simulink model "simulink_Pcontroller"  (R2016a)
settings: Solver=ode1  StartTime=0.0  StopTime=inf  FixedStep=0.1  RelTol=1e-3
undefined symbols (not defined in the file): serial
libraries: instrumentlib x4, simulink x2, dspswit3 x1
settings Model: Creator=Andrei  LastModifiedBy=Andrei

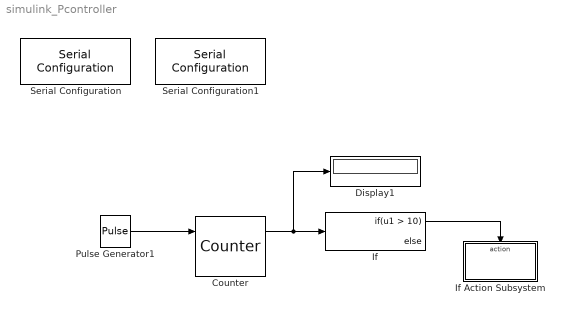
== system simulink_Pcontroller ==
  Counter : dspswit3/Counter  Direction=Up  CountEvent=Falling edge  CounterSize=8 bits  MaxCount=255  InitialCount=0  Output=Count and Hit  HitValue=32  ResetInput=on  SamplesPerFrame=1  Ts=1  CntDtype=uint8  HitDtype=Logical
  Display1 : Display
  If : If  IfExpression=u1 > 10
  If Action Subsystem : Subsystem  TreatAsAtomicUnit=on
  Pulse Generator1 : DiscretePulseGenerator  PulseType=Time based  Period=500  PulseWidth=50
  Serial Configuration : instrumentlib/Serial Configuration  Priority=-200000  ComPortMenu=COM5  ComPort=COM5  ObjConstructor=serial('COM5');  BaudRate=9600  DataBits=8  Parity=none  StopBits=1  FlowControl=none  Timeout=10  ByteOrder=LittleEndian
  Serial Configuration1 : instrumentlib/Serial Configuration  Priority=-200000  ComPortMenu=COM3  ComPort=COM3  ObjConstructor=serial('COM3');  BaudRate=38400  DataBits=8  Parity=none  StopBits=1  FlowControl=none  Timeout=10  ByteOrder=LittleEndian
  wires:
  Counter/1 -> Display1/1, If/1
  Pulse Generator1/1 -> Counter/1
  If/1 -> If Action Subsystem/Action

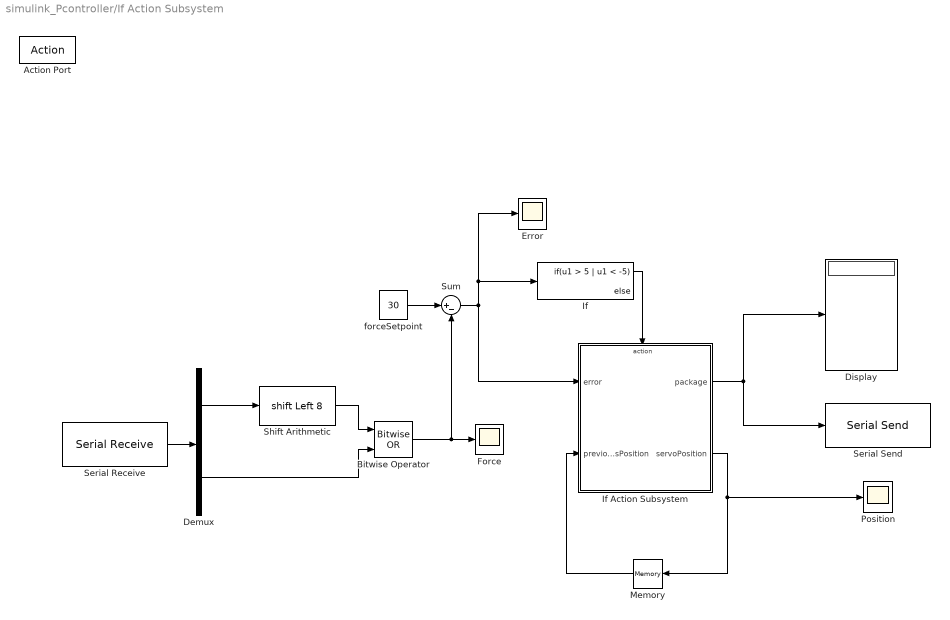
== system simulink_Pcontroller/If Action Subsystem ==
  Action Port : ActionPort  ActionType=then
  Bitwise Operator : simulink/Logic and Bit Operations/Bitwise Operator  logicop=OR  UseBitMask=off  NumInputPorts=2  BitMask=bin2dec('11011001')  BitMaskRealWorld=Stored Integer
  Demux : Demux  Outputs=2
  Display : Display
  "Error " : Scope
  Force : Scope
  If : If  IfExpression=u1 > 5 | u1 < -5
  If Action Subsystem : Subsystem  TreatAsAtomicUnit=on
  Memory : Memory  X0=512  InheritSampleTime=on
  "Position " : Scope
  Serial Receive : instrumentlib/Serial Receive  ComPortMenu=COM5  ComPort=COM5  ObjConstructor=serial('COM5');  Header=$  Terminator=!  DataSize="[1  2]"  DataType=uint8  EnableBlockingMode=on  ActionDataUnavailable=Output last received value  CustomValue=0  SampleTime=0.1
  Serial Send : instrumentlib/Serial Send  ComPortMenu=COM3  ComPort=COM3  ObjConstructor=serial('COM3');  Terminator=<none>  EnableBlockingMode=on
  Shift Arithmetic : ArithShift  BitShiftNumber=8  BitShiftDirection=Left
  Sum : Sum  Inputs=|+-
  forceSetpoint : Constant  Value=30
  wires:
  Serial Receive/1 -> Demux/1
  Demux/1 -> Shift Arithmetic/1
  Shift Arithmetic/1 -> Bitwise Operator/1
  Demux/2 -> Bitwise Operator/2
  Bitwise Operator/1 -> Force/1, Sum/2
  forceSetpoint/1 -> Sum/1
  Sum/1 -> "Error "/1, If/1, If Action Subsystem/1(error)
  If/1 -> If Action Subsystem/Action
  If Action Subsystem/1(package) -> Display/1, Serial Send/1
  If Action Subsystem/2(servoPosition) -> "Position "/1, Memory/1
  Memory/1 -> If Action Subsystem/2(previousPosition)

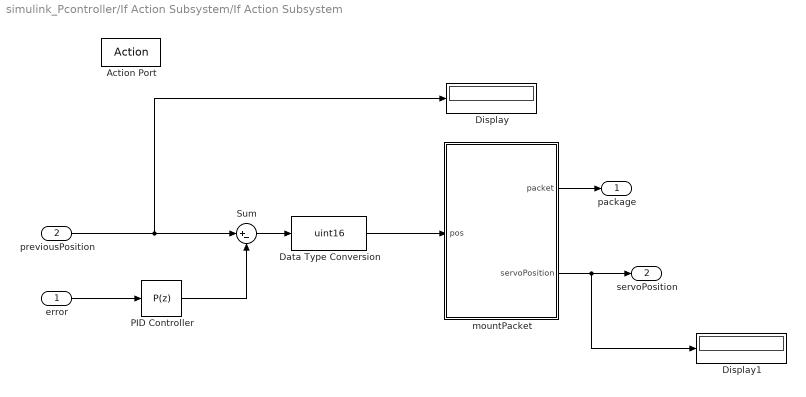
== system simulink_Pcontroller/If Action Subsystem/If Action Subsystem ==
  error : Inport
  previousPosition : Inport  Port=2
  Action Port : ActionPort  ActionType=then
  Data Type Conversion : DataTypeConversion  OutDataTypeStr=uint16
  Display : Display
  Display1 : Display
  PID Controller : simulink/Continuous/PID Controller  Controller=P  TimeDomain=Discrete-time  SampleTime=-1  IntegratorMethod=Forward Euler  FilterMethod=Forward Euler  Form=Parallel  UseFilter=on  ControllerParametersSource=internal  P=0.3  I=1  D=0  N=100  InitialConditionSource=internal  InitialConditionForIntegrator=0  InitialConditionForFilter=0  ExternalReset=none  LimitOutput=on  UpperSaturationLimit=512  LowerSaturationLimit=0  LinearizeAsGain=on  AntiWindupMode=none  Kb=1  TrackingMode=off  Kt=1  PParamMin=[]  PParamMax=[]  PParamDataTypeStr=double  IParamMin=[]  IParamMax=[]  DParamMin=[]  DParamMax=[]  NParamMin=[]  NParamMax=[]  KbParamMin=[]  KbParamMax=[]  KtParamMin=[]  KtParamMax=[]  POutMin=[]  POutMax=[]  POutDataTypeStr=double  PGainOutDataTypeStr=double  PProdOutDataTypeStr=double  IOutMin=[]  IOutMax=[]  DOutMin=[]  DOutMax=[]  NOutMin=[]  NOutMax=[]  KbOutMin=[]  KbOutMax=[]  KtOutMin=[]  KtOutMax=[]  IntegratorOutMin=[]  IntegratorOutMax=[]  FilterOutMin=[]  FilterOutMax=[]  SumOutMin=[]  SumOutMax=[]  SumI1OutMin=[]  SumI1OutMax=[]  SumI2OutMin=[]  SumI2OutMax=[]  SumI3OutMin=[]  SumI3OutMax=[]  SumDOutMin=[]  SumDOutMax=[]  SaturationOutMin=[]  SaturationOutMax=[]  SaturationOutDataTypeStr=uint16  IntegratorContinuousStateAttributes=''  IntegratorStateMustResolveToSignalObject=off  IntegratorRTWStateStorageClass=Auto  FilterContinuousStateAttributes=''  FilterStateMustResolveToSignalObject=off  FilterRTWStateStorageClass=Auto  DifferentiatorICPrevScaledInput=0  DifferentiatorOutMin=[]  DifferentiatorOutMax=[]
  Sum : Sum  Inputs=|+-
  mountPacket : MATLAB Function  TreatAsAtomicUnit=on
  package : Outport
  servoPosition : Outport  Port=2
  wires:
  error/1 -> PID Controller/1
  mountPacket/1(packet) -> package/1
  mountPacket/2(servoPosition) -> Display1/1, servoPosition/1
  Data Type Conversion/1 -> mountPacket/1(pos)
  Sum/1 -> Data Type Conversion/1
  PID Controller/1 -> Sum/2
  previousPosition/1 -> Display/1, Sum/1

== matlab function simulink_Pcontroller/If Action Subsystem/If Action Subsystem/mountPacket ==
  data: pos input; packet output; servoPosition output
function [packet,servoPosition] = sendSerialData(pos)     
    posMSB = uint8(bitshift(pos,-8)); %equivalent to pos>>8
    posLSB = uint8(bitand(pos,255)); %equivalent to pos&0XFF
    packet = uint8(zeros(1,6));
    servoPosition = pos;
    packet(1) = uint8(36); %header: '$'
    packet(2) = uint8(0); %action
    packet(3) = uint8(6); %servo
    packet(4) = uint8(posMSB); %posMSB
    packet(5) = uint8(posLSB); %posLSB
    packet(6) = uint8(33); %end package: '!'
    packet = uint8(packet);
end
